simulink model "sim01"  (R2023b)
settings: Solver=VariableStepAuto  StartTime=0.0  StopTime=10.0  RelTol=1e-3
values from neighbouring files (symbols this model uses):
  A = [-1 5;0 -8]    [es1.m]
  B = [1 0]'    [es1.m]
  C = [1 5]    [es1.m]
  ueq = 3    [es1.m]
  x0 = 0    [es1.m]
settings Model: Creator=stefa  LastModifiedBy=stefa
settings OptimizationCC: ReuseModelBlockBuffer=off

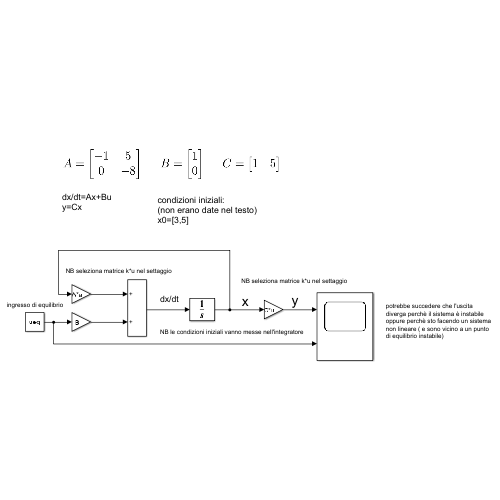
[thumbnail: Simulink's stored preview of the top-level diagram]
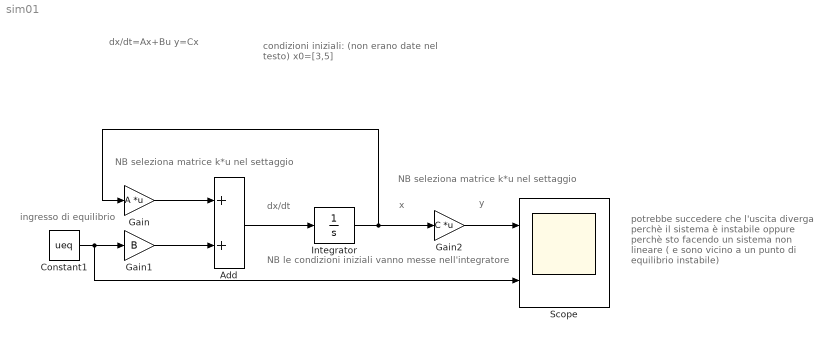
== system sim01 ==
  note: ingresso di equilibrio
  note: potrebbe succedere che l'uscita diverga perchè il sistema è instabile oppure perchè sto facendo un sistema non lineare ( e sono vicino a un punto di equilibrio instabile)
  note: NB le condizioni iniziali vanno messe nell'integratore
  note: condizioni iniziali:
      | (non erano date nel testo)
      | x0=[3,5]
  note: NB seleziona matrice k*u nel settaggio
  note: y
  note: dx/dt=Ax+Bu
      | y=Cx
  note: x
  note: dx/dt
  note: NB seleziona matrice k*u nel settaggio
  Add : Sum
  Constant1 : Constant  Value=ueq
  Gain : Gain  Gain=A  Multiplication=Matrix(K*u)
  Gain1 : Gain  Gain=B
  Gain2 : Gain  Gain=C  Multiplication=Matrix(K*u)
  Integrator : Integrator  InitialCondition=x0
  Scope : Scope  NumInputPorts=2
  wires:
  Constant1/1 -> Scope/2, Gain1/1
  Gain1/1 -> Add/2
  Gain/1 -> Add/1
  Add/1 -> Integrator/1
  Integrator/1 -> Gain2/1, Gain/1
  Gain2/1 -> Scope/1
